simulink model "PMSM_MPCC"  (R2022b)
settings: Solver=FixedStepDiscrete  StartTime=0.0  StopTime=0.5  FixedStep=1e-6  RelTol=1e-3
model workspace (MAT data in the model file):
  B = 0
  Current_Filter_On = 0
  F = 10000
  J = 5.8e-05
  Ls = 0.0005125
  Pn = 5
  Rs = 0.1445
  T = 0.0001
  T_deadband = 3e-06
  Ts = 5e-05
  Vdc = 60
  psi_f = 0.0113
  speed_ki = 1.2
  speed_kp = 0.7
undefined symbols (not defined in the file): sigbuilder_block
libraries: spsDCVoltageSourceLib x1, dspstat3 x1, spsPermanentMagnetSynchronousMachineLib x1, slpidlib x1, spsTwoLevelConverterLib x1, spspowerguiLib x1, simulink x1
(part 2 of 2)

== matlab function PMSM_MPCC/MPCC/MATLAB Function ==
  data: index input; Ua output; Ub output; Uc output
function [Ua,Ub,Uc] = fcn(index)
switch index
    case 0
        Ua=0;
        Ub=0;
        Uc=0;
    case 1
        Ua=0;
        Ub=0;
        Uc=1;
    case 2
        Ua=0;
        Ub=1;
        Uc=0;
    case 3
        Ua=0;
        Ub=1;
        Uc=1;
    case 4
        Ua=1;
        Ub=0;
        Uc=0;
    case 5
        Ua=1;
        Ub=0;
        Uc=1;
    case 6
        Ua=1;
        Ub=1;
        Uc=0;
    case 7
        Ua=1;
        Ub=1;
        Uc=1;
    otherwise
        Ua=0;
        Ub=0;
        Uc=0;
end

== matlab function PMSM_MPCC/MPCC/Subsystem/MATLAB Function1 ==
  data: T input; id_k_2 output; Rs input; Ls input; we input; id_k_1 input; iq_k_1 input; ud_k_1 input; uq_k_1 input; iq_k_2 output; psi_f input
function [id_k_2,iq_k_2] = fcn(T,Rs,Ls,we,id_k_1,iq_k_1,ud_k_1,uq_k_1,psi_f)

id_k_2 = (1-T*Rs/Ls)*id_k_1+T/Ls*ud_k_1+T*we*iq_k_1;
iq_k_2 = (1-T*Rs/Ls)*iq_k_1+T/Ls*uq_k_1-T*we*id_k_1-T*we*psi_f/Ls;

== matlab function PMSM_MPCC/MPCC/Subsystem1/MATLAB Function ==
  data: T input; id_k_1 output; Rs input; Ls input; we input; id_k input; iq_k input; ud_k input; uq_k input; iq_k_1 output; psi_f input
function [id_k_1,iq_k_1] = fcn(T,Rs,Ls,we,id_k,iq_k,ud_k,uq_k,psi_f)

id_k_1 = (1-T*Rs/Ls)*id_k+T/Ls*ud_k+T*we*iq_k;
iq_k_1 = (1-T*Rs/Ls)*iq_k+T/Ls*uq_k-T*we*id_k-T*we*psi_f/Ls;

== matlab function PMSM_MPCC/MPCC/Subsystem1/MATLAB Function1 ==
  data: T input; id_k_2 output; Rs input; Ls input; we input; id_k_1 input; iq_k_1 input; ud_k_1 input; uq_k_1 input; iq_k_2 output; psi_f input
function [id_k_2,iq_k_2] = fcn(T,Rs,Ls,we,id_k_1,iq_k_1,ud_k_1,uq_k_1,psi_f)

id_k_2 = (1-T*Rs/Ls)*id_k_1+T/Ls*ud_k_1+T*we*iq_k_1;
iq_k_2 = (1-T*Rs/Ls)*iq_k_1+T/Ls*uq_k_1-T*we*id_k_1-T*we*psi_f/Ls;

== matlab function PMSM_MPCC/MPCC/Subsystem2/MATLAB Function ==
  data: T input; id_k_1 output; Rs input; Ls input; we input; id_k input; iq_k input; ud_k input; uq_k input; iq_k_1 output; psi_f input
function [id_k_1,iq_k_1] = fcn(T,Rs,Ls,we,id_k,iq_k,ud_k,uq_k,psi_f)

id_k_1 = (1-T*Rs/Ls)*id_k+T/Ls*ud_k+T*we*iq_k;
iq_k_1 = (1-T*Rs/Ls)*iq_k+T/Ls*uq_k-T*we*id_k-T*we*psi_f/Ls;
